simulink model "dianping3"  (R2016a)
settings: Solver=VariableStepAuto  StartTime=0.0  StopTime=1  RelTol=1e-3
libraries: powerlib x12, powerlib_meascontrol x1, dspstat3 x1
settings Model: Creator=24535  LastModifiedBy=24535

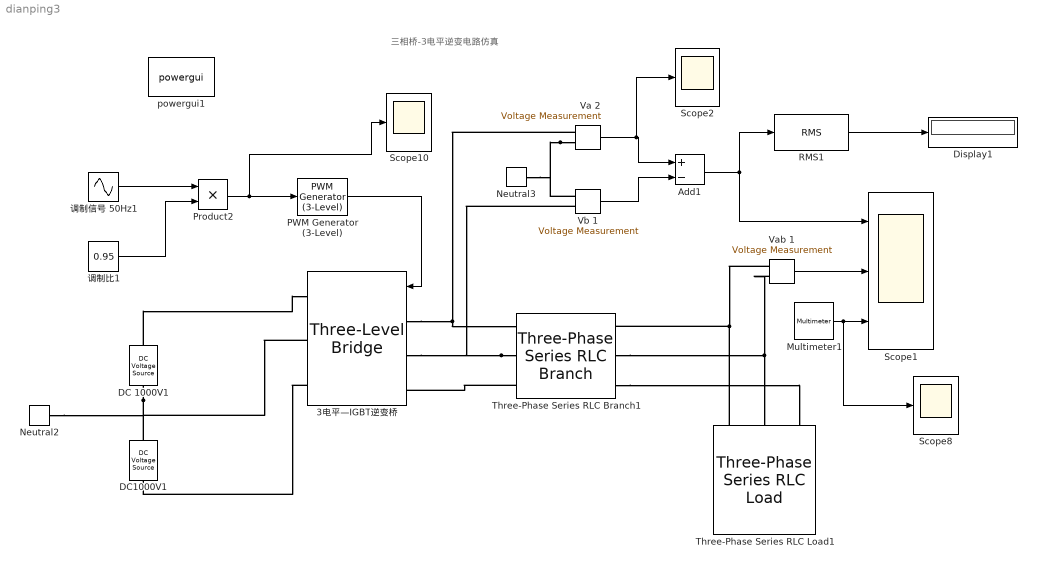
== system dianping3 ==
  note: 三相桥-3电平逆变电路仿真
  3电平—IGBT逆变桥 : powerlib/Power Electronics/Three-Level Bridge  Arms=3  SnubberResistance=1e5  SbubberCapacitance=inf  Device=IGBT / Diodes  Ron=1e-3  ForwardVoltages="[  0  0  ]"  Measurements=None
  Add1 : Sum  Inputs=+-
  DC 1000V1 : powerlib/Electrical Sources/DC Voltage Source  Amplitude=1000  Measurements=None
  DC1000V1 : powerlib/Electrical Sources/DC Voltage Source  Amplitude=1000  Measurements=None
  Display1 : Display
      settings: Decimation=100
  Multimeter1 : powerlib/Measurements/Multimeter  PhasorSimulation=off  OutputType=Complex  sel=4  L=6  Gain=1  yselected={'Iag: Three-Phase Series RLC Load1'};  PSBOutputType=1  PSBequivalent=0  AxesSetting=[0,0.1,-100,100]  Display=0  SavedBlockNames=-11
  Neutral2 : powerlib/Elements/Neutral  LConnTagsString=a  NodeNumber=1
  Neutral3 : powerlib/Elements/Neutral  LConnTagsString=a  NodeNumber=1
  PWM Generator (3-Level) : powerlib_meascontrol/Pulse & Signal Generators/PWM Generator (3-Level)  ModulatorType=Three-phase bridge (12 pulses)  ModulatorMode=Unsynchronized  nF=27  Fc=33*50  ModulatingSignals=off  m=0.8  Freq=60  Phase=0  Ts=0
  Product2 : Product
  RMS1 : dspstat3/RMS  run=off  reset_popup=None  InputProcessing=Columns as channels (frame based)  directionMode=Each column  dimension=1
  Scope1 : Scope  NumInputPorts=3
  Scope10 : Scope
  Scope2 : Scope
  Scope8 : Scope
  Three-Phase Series RLC Branch1 : powerlib/Elements/Three-Phase Series RLC Branch  LConnTagsString=A|B|C  RConnTagsString=A|B|C  BranchType=RL  Resistance=10e-3  Inductance=100e-6  Capacitance=1e-6  Measurements=None
  Three-Phase Series RLC Load1 : powerlib/Elements/Three-Phase Series RLC Load  LConnTagsString=A|B|C  Configuration=Y (grounded)  NominalVoltage=2000  Vabc=[1e3 1e3 1e3]  Vabcp=[1e3 1e3 1e3]  NominalFrequency=50  UnbalancedPower=off  ActivePower=500e3  InductivePower=100e3  CapacitivePower=0  Pabc=[10e3 9e3 11e3]  QLabc=[100 90 110]  QCabc=[100 90 110]  Pabcp=[10e3 9e3 11e3]  QLabcp=[100 90 110]  QCabcp=[100 90 110]  Measurements=Branch voltages and currents  LoadType=constant Z
  Va 2 : powerlib/Measurements/Voltage Measurement  PhasorSimulation=off  OutputType=Complex  PSBequivalent=0
  Vab 1 : powerlib/Measurements/Voltage Measurement  PhasorSimulation=off  OutputType=Complex  PSBequivalent=0
  Vb 1 : powerlib/Measurements/Voltage Measurement  PhasorSimulation=off  OutputType=Complex  PSBequivalent=0
  powergui1 : powerlib/powergui  Priority=1  SimulationMode=Discrete  SolverType=Tustin/Backward Euler (TBE)  SampleTime=2e-6  frequency=60  SPID=off  DisableSnubberDevices=off  DisableRonSwitches=off  DisableVfSwitches=off  SwTol=0  DisplayEquations=off  Interpol=off  ExternalGateDelay=off  methode=off  Ts=10  FunctionMessages=off  echomessages=off  HookPort=off  EnableUseOfTLC=off  x0status=blocks  frequencyindice=0  Pbase=100e6  ErrMax=1e-4  Iterations=50  UnitsV=kV  UnitsW=MW  buscounter=0  RestoreLinks=warning  ResistiveCurrentMeasurement=off  Frange=[0:2:500]  Ylog=off  Xlog=on  ShowGrid=off  save=off  variable=ZData  structure=level33  ZoomFFT=off  StartTime=0.0  cycles=4  DisplayStyle=1  fundamental=50  FreqAxis=off  MaxFrequency=6000  frequencyindicesteady=1  RmsSteady=1  display=off
  调制信号 50Hz1 : Sin  Frequency=100*pi  Phase=[0 -2*pi/3 2*pi/3]  SampleTime=0
  调制比1 : Constant  Value=0.95
  wires:
  调制信号 50Hz1/1 -> Product2/1
  调制比1/1 -> Product2/2
  Product2/1 -> PWM Generator (3-Level)/1, Scope10/1
  PWM Generator (3-Level)/1 -> 3电平—IGBT逆变桥/1
  Multimeter1/1 -> Scope8/1, Scope1/3
  Vab 1/1 -> Scope1/2
  RMS1/1 -> Display1/1
  Va 2/1 -> Scope2/1, Add1/1
  Vb 1/1 -> Add1/2
  Add1/1 -> Scope1/1, RMS1/1
  connections:
  DC 1000V1/LConn1 -- 3电平—IGBT逆变桥/RConn2 -- DC1000V1/RConn1 -- Neutral2/LConn1
  Va 2/LConn1 -- 3电平—IGBT逆变桥/LConn1 -- Three-Phase Series RLC Branch1/LConn1
  Three-Phase Series RLC Branch1/LConn2 -- 3电平—IGBT逆变桥/LConn2 -- Vb 1/LConn1
  Vab 1/LConn1 -- Three-Phase Series RLC Load1/LConn1 -- Three-Phase Series RLC Branch1/RConn1
  Vab 1/LConn2 -- Three-Phase Series RLC Branch1/RConn2 -- Three-Phase Series RLC Load1/LConn2
  Va 2/LConn2 -- Neutral3/LConn1 -- Vb 1/LConn2
  Three-Phase Series RLC Branch1/RConn3 -- Three-Phase Series RLC Load1/LConn3
  Three-Phase Series RLC Branch1/LConn3 -- 3电平—IGBT逆变桥/LConn3
  DC 1000V1/RConn1 -- 3电平—IGBT逆变桥/RConn1
  3电平—IGBT逆变桥/RConn3 -- DC1000V1/LConn1
